simulink model "foc"  (R2024b)
settings: Solver=VariableStepAuto  StartTime=0.0  StopTime=3  RelTol=1e-3
values from neighbouring files (symbols this model uses):
  pmsm =     [foc.mat]    (also in inverter.mat; speed_control.mat; vbyf.mat)
  Ts = 2.5e-05    [foc.mat]    (also in inverter.mat; speed_control.mat; vbyf.mat)
libraries: mcbcontrollergainlib x2, mcbfoclib x1, mcbpositiondecoderlib x1, mcbplantlib x1, autolibpmsminterior x1, slpidlib x1
settings Model: Creator=realf  LastModifiedBy=realf

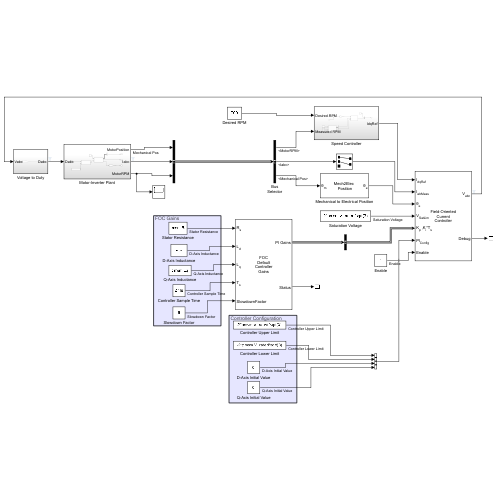
[thumbnail: Simulink's stored preview of the top-level diagram]
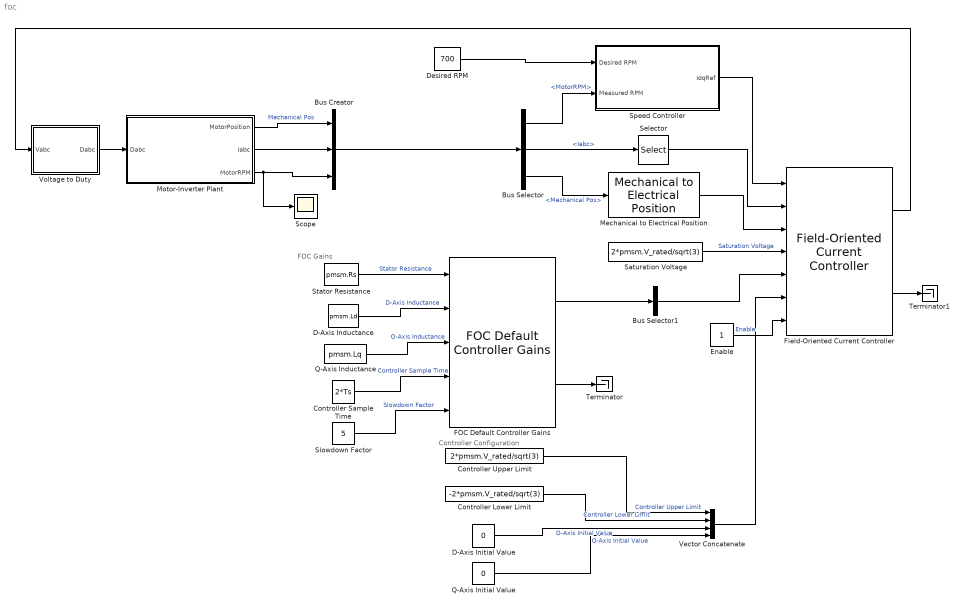
== system foc ==
  note: Controller Configuration
  note: FOC Gains
  Bus Creator : BusCreator  Inputs=3
  Bus Selector : BusSelector  OutputSignals=MotorRPM,Iabc,Mechanical Pos
  Bus Selector1 : BusSelector  OutputSignals=Daxis_Kp,Daxis_Ki*Ts,Qaxis_Kp,Qaxis_Ki*Ts  OutputAsBus=on
  Controller Lower Limit : Constant  Value=-2*pmsm.V_rated/sqrt(3)
  Controller Sample Time : Constant  Value=2*Ts
  Controller Upper Limit : Constant  Value=2*pmsm.V_rated/sqrt(3)  OutDataTypeStr=double
  D-Axis Inductance : Constant  Value=pmsm.Ld
  D-Axis Initial Value : Constant  Value=0
  Desired RPM : Constant  Value=700
  Enable : Constant
  FOC Default Controller Gains : mcbcontrollergainlib/FOC Default Controller Gains  motorSelection=PMSM  unitType=SI Unit  outCurrentControlGain=on  outFWCGain=off  outSpeedControlGain=off  externalDelay=off  currentSensorDelay=50e-6  speedSensorDelay=50e-6  speedFilterDelay=0.02
      settings: LibrarySourceBlock=mcblib/Controls/Controllers/FOC Default Controller Gains
  Field-Oriented Current Controller : mcbfoclib/Field-Oriented Current Controller  AngleUnit=Radians  NumberOfLUTPoints=1024  AxisAlignment=D-axis  SaturationMethod=D-Q equivalence  PWMMethod=SVM: space vector modulation
      settings: LibrarySourceBlock=mcblib/Controls/Controllers/Field-Oriented Current Controller
  Mechanical to Electrical Position : mcbpositiondecoderlib/Mechanical to Electrical Position  PolePairsInputType=Specify via dialog  NrPP=pmsm.p  selectedRange=Radians  MechOfstInputType=Specify via dialog  mechOffsetIn=0  maxAngleIn=2*pi  InputDataType=single  VariantSelect=floating-point
      settings: LibrarySourceBlock=mcblib/Sensor Decoders/Mechanical to Electrical Position
  Motor-Inverter Plant : Subsystem
  Q-Axis Inductance : Constant  Value=pmsm.Lq
  Q-Axis Initial Value : Constant  Value=0
  Saturation Voltage : Constant  Value=2*pmsm.V_rated/sqrt(3)
  Scope : Scope
  Selector : Selector  InputPortWidth=3  IndexOptions=Index vector (dialog)  Indices=[1 2]  OutputSizes=1
  Slowdown Factor : Constant  Value=5
  Speed Controller : Subsystem
  Stator Resistance : Constant  Value=pmsm.Rs
  Terminator : Terminator
  Terminator1 : Terminator
  Vector Concatenate : Concatenate  NumInputs=4
  Voltage to Duty : Subsystem
  wires:
  Field-Oriented Current Controller/2 -> Terminator1/1
  Field-Oriented Current Controller/1 -> Voltage to Duty/1(Vabc)
  Bus Selector1/1 -> Field-Oriented Current Controller/5
  Voltage to Duty/1(Dabc) -> Motor-Inverter Plant/1(Dabc)
  Motor-Inverter Plant/1(MotorPosition) -> Bus Creator/1  "Mechanical Pos"
  Motor-Inverter Plant/3(MotorRPM) -> Bus Creator/3, Scope/1
  Motor-Inverter Plant/2(Iabc) -> Bus Creator/2
  Bus Creator/1 -> Bus Selector/1
  Enable/1 -> Field-Oriented Current Controller/7  "Enable"
  Speed Controller/1(IdqRef) -> Field-Oriented Current Controller/1
  Bus Selector/3 -> Mechanical to Electrical Position/1  "<Mechanical Pos>"
  Bus Selector/2 -> Selector/1  "<Iabc>"
  Bus Selector/1 -> Speed Controller/2(Measured RPM)  "<MotorRPM>"
  FOC Default Controller Gains/1 -> Bus Selector1/1
  FOC Default Controller Gains/2 -> Terminator/1
  Saturation Voltage/1 -> Field-Oriented Current Controller/4  "Saturation Voltage"
  Selector/1 -> Field-Oriented Current Controller/2
  Mechanical to Electrical Position/1 -> Field-Oriented Current Controller/3
  Vector Concatenate/1 -> Field-Oriented Current Controller/6
  D-Axis Initial Value/1 -> Vector Concatenate/3  "D-Axis Initial Value"
  D-Axis Inductance/1 -> FOC Default Controller Gains/2  "D-Axis Inductance"
  Q-Axis Inductance/1 -> FOC Default Controller Gains/3  "Q-Axis Inductance"
  Q-Axis Initial Value/1 -> Vector Concatenate/4  "Q-Axis Initial Value"
  Stator Resistance/1 -> FOC Default Controller Gains/1  "Stator Resistance"
  Slowdown Factor/1 -> FOC Default Controller Gains/5  "Slowdown Factor"
  Controller Sample Time/1 -> FOC Default Controller Gains/4  "Controller Sample Time"
  Controller Upper Limit/1 -> Vector Concatenate/1  "Controller Upper Limit"
  Controller Lower Limit/1 -> Vector Concatenate/2  "Controller Lower Limit"
  Desired RPM/1 -> Speed Controller/1(Desired RPM)

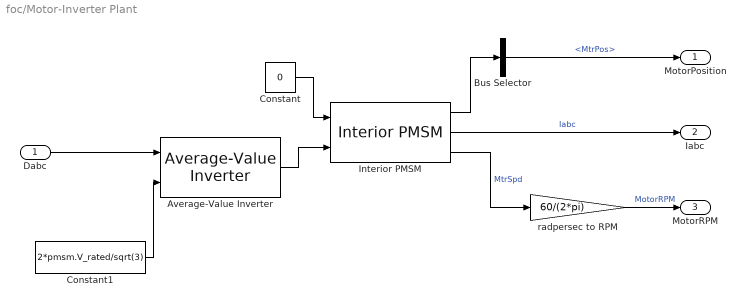
== system foc/Motor-Inverter Plant ==
  Dabc : Inport
  Average-Value Inverter : mcbplantlib/Average-Value Inverter
  Bus Selector : BusSelector  OutputSignals=MtrPos
  Constant : Constant  Value=0
  Constant1 : Constant  Value=2*pmsm.V_rated/sqrt(3)
  Interior PMSM : autolibpmsminterior/Interior PMSM  port_config=Torque  sim_type=Discrete  Ts=Ts  P=pmsm.p  Rs=pmsm.Rs  Ldq=[pmsm.Ld, pmsm.Lq]  KConstText=Permanent flux linkage constant (lambda_pm):  lambda_pm=pmsm.FluxPM  Ke=159.9771  mechanical=[pmsm.J, 0, 0]  idq0=[0 0]  theta_init=0  omega_init=0  KConst=pmsm.FluxPM  lambda_pm_calc=pmsm.FluxPM  Kt=0.07  RefBlkName='autolibpmsminterior/Interior PMSM'  aMode=5
  radpersec to RPM : Gain  Gain=60/(2*pi)
  MotorPosition : Outport
  Iabc : Outport  Port=2
  MotorRPM : Outport  Port=3
  wires:
  Interior PMSM/3 -> radpersec to RPM/1  "MtrSpd"
  Interior PMSM/2 -> Iabc/1  "Iabc"
  Average-Value Inverter/1 -> Interior PMSM/2
  Interior PMSM/1 -> Bus Selector/1
  Bus Selector/1 -> MotorPosition/1  "<MtrPos>"
  Constant1/1 -> Average-Value Inverter/2
  Constant/1 -> Interior PMSM/1
  Dabc/1 -> Average-Value Inverter/1
  radpersec to RPM/1 -> MotorRPM/1  "MotorRPM"

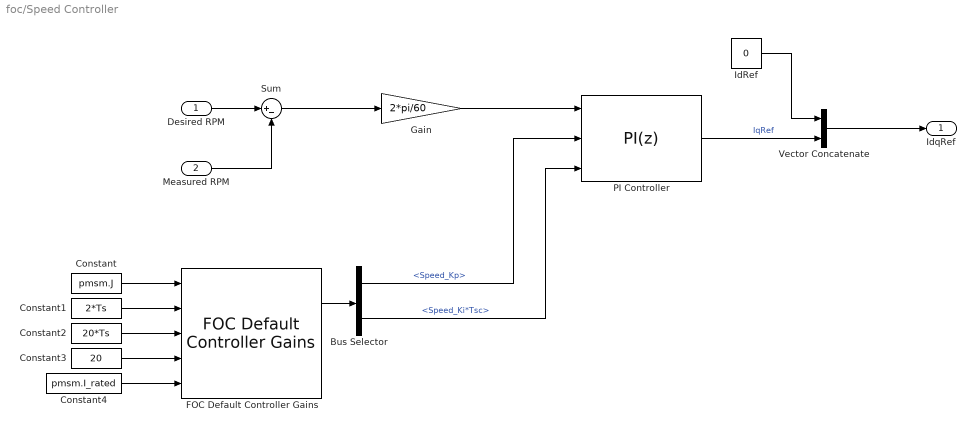
== system foc/Speed Controller ==
  Desired RPM : Inport
  Measured RPM : Inport  Port=2
  Bus Selector : BusSelector  OutputSignals=Speed_Kp,Speed_Ki*Tsc
  Constant : Constant  Value=pmsm.J
  Constant1 : Constant  Value=2*Ts
  Constant2 : Constant  Value=20*Ts
  Constant3 : Constant  Value=20
  Constant4 : Constant  Value=pmsm.I_rated
  FOC Default Controller Gains : mcbcontrollergainlib/FOC Default Controller Gains  motorSelection=PMSM  unitType=SI Unit  outCurrentControlGain=off  outFWCGain=off  outSpeedControlGain=on  externalDelay=off  currentSensorDelay=50e-6  speedSensorDelay=50e-6  speedFilterDelay=0.02
  Gain : Gain  Gain=2*pi/60
  IdRef : Constant  Value=0
  PI Controller : slpidlib/PID Controller  Controller=PI  Form=Parallel  TimeDomain=Discrete-time  UseExternalTs=off  SampleTime=-1  IntegratorMethod=Forward Euler  FilterMethod=Forward Euler  ControllerParametersSource=external  P=1  I=1  UseKiTs=on  D=0  UseExternalDerivativeSource=off  N=100  UseFilter=on  TunerSelectOption=Transfer Function Based (PID Tuner App)  InitialConditionSource=internal  InitialConditionForIntegrator=0  InitialConditionForFilter=0  DifferentiatorICPrevScaledInput=0  ExternalReset=none  TrackingMode=off  Kt=1  LimitOutput=on  SatLimitsSource=internal  UpperSaturationLimit=pmsm.I_rated  LowerSaturationLimit=-pmsm.I_rated  LinearizeAsGain=on  AntiWindupMode=clamping  Kb=1  LimitIntegrator=on  UpperIntegratorSaturationLimit=pmsm.I_rated  LowerIntegratorSaturationLimit=-pmsm.I_rated  RndMeth=Simplest  POutMin=[]  POutMax=[]  IOutMin=[]  IOutMax=[]  DOutMin=[]  DOutMax=[]  NOutMin=[]  NOutMax=[]  SumOutMin=[]  SumOutMax=[]  SaturationOutDataTypeStr=Inherit: Inherit via back propagation  SaturationOutMin=[]  SaturationOutMax=[]  PParamMin=[]  PParamMax=[]  IParamMin=[]  IParamMax=[]  DParamMin=[]  DParamMax=[]  NParamMin=[]  NParamMax=[]  KbParamMin=[]  KbParamMax=[]  KtParamMin=[]  KtParamMax=[]  KbOutMin=[]  KbOutMax=[]  KtOutMin=[]  KtOutMax=[]  IntegratorOutMin=[]  IntegratorOutMax=[]  FilterOutMin=[]  FilterOutMax=[]  SumI1OutMin=[]  SumI1OutMax=[]  SumI2OutMin=[]  SumI2OutMax=[]  SumI3OutMin=[]  SumI3OutMax=[]  SumI4OutMin=[]  SumI4OutMax=[]  SumDOutMin=[]  SumDOutMax=[]  DifferentiatorOutMin=[]  DifferentiatorOutMax=[]  FilterDiffOutCoefMin=[]  FilterDiffOutCoefMax=[]  ReciprocalOutMin=[]  ReciprocalOutMax=[]  SumDenOutMin=[]  SumDenOutMax=[]  SumNumOutMin=[]  SumNumOutMax=[]  DivideOutMin=[]  DivideOutMax=[]  UdiffTsProdOutMin=[]  UdiffTsProdOutMax=[]  NTsProdOutMin=[]  NTsProdOutMax=[]  UintegralTsProdOutMin=[]  UintegralTsProdOutMax=[]  UngainTsProdOutMin=[]  UngainTsProdOutMax=[]  ClampingZeroOutDataTypeStr=Inherit: Inherit via back propagation  ClampingZeroOutMin=[]  ClampingZeroOutMax=[]  FilterDenConstantOutDataTypeStr=Inherit: Inherit via back propagation  FilterDenConstantOutMin=[]  FilterDenConstantOutMax=[]  PCopyOutDataTypeStr=Inherit: Inherit via back propagation  PCopyOutMin=[]  PCopyOutMax=[]  NCopyOutDataTypeStr=Inherit: Inherit via back propagation  NCopyOutMin=[]  NCopyOutMax=[]  IntegratorContinuousStateAttributes=''  IntegratorStateMustResolveToSignalObject=off  IntegratorRTWStateStorageClass=Auto  FilterContinuousStateAttributes=''  FilterStateMustResolveToSignalObject=off  FilterRTWStateStorageClass=Auto  ParallelPVariant=ExternalParameters  IdealPVariant=Disabled  IVariant=ExternalParameters  DVariant=Disabled  IntegratorVariant=Discrete  SatVariant=Enabled  AWVariant=DiscClampingParallel  PCopyVariant=Disabled  TRVariant=Disabled  FdbkBlocksVariant=Forward  IdealPFdbkVariant=Disabled  SatFdbkVariant=Disabled  DerivativeFilterVariant=Disabled  NVariant=Disabled  NCopyVariant=Disabled_SignalSpec  FilterICVariant=Disabled  IntegratorICVariant=InternalICs  ExternalResetVariant=Disabled  TRSumVariant=Passthrough  SumFdbkVariant=Disabled  SumVariant=Sum_PI  TsampFilterVariant=InternalTs  TsampNgainVariant=Passthrough  TsampIntegralVariant=Disabled_SignalSpec  ExternalSaturationOutDataTypeStr=Inherit: Same as second input  DerivativeSourceVariant=Disabled  PreIntVariant=InternalPreInt
  Sum : Sum  Inputs=|+-
  Vector Concatenate : Concatenate
  IdqRef : Outport
  wires:
  Gain/1 -> PI Controller/1
  IdRef/1 -> Vector Concatenate/1
  Vector Concatenate/1 -> IdqRef/1
  PI Controller/1 -> Vector Concatenate/2  "IqRef"
  Bus Selector/2 -> PI Controller/3  "<Speed_Ki*Tsc>"
  Bus Selector/1 -> PI Controller/2  "<Speed_Kp>"
  FOC Default Controller Gains/1 -> Bus Selector/1
  Constant4/1 -> FOC Default Controller Gains/5
  Constant3/1 -> FOC Default Controller Gains/4
  Constant2/1 -> FOC Default Controller Gains/3
  Constant1/1 -> FOC Default Controller Gains/2
  Constant/1 -> FOC Default Controller Gains/1
  Sum/1 -> Gain/1
  Measured RPM/1 -> Sum/2
  Desired RPM/1 -> Sum/1

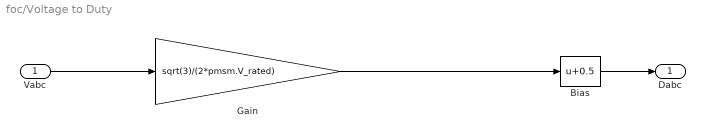
== system foc/Voltage to Duty ==
  Vabc : Inport
  Bias : Bias  Bias=0.5  SaturateOnIntegerOverflow=off
  Gain : Gain  Gain=sqrt(3)/(2*pmsm.V_rated)
  Dabc : Outport
  wires:
  Gain/1 -> Bias/1
  Bias/1 -> Dabc/1
  Vabc/1 -> Gain/1
